simulink model "TZ"  (R2023a)
settings: Solver=VariableStepAuto  StartTime=0.0  StopTime=25.0  RelTol=1e-3
settings Model: Creator=zarok  LastModifiedBy=Georgiy

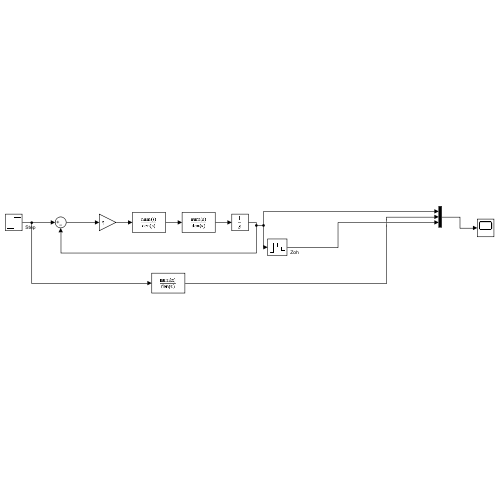
[thumbnail: Simulink's stored preview of the top-level diagram]
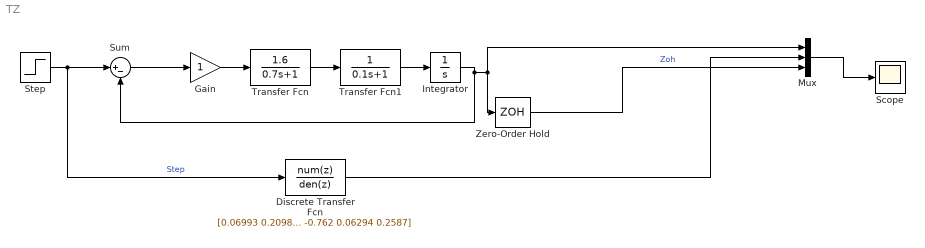
== system TZ ==
  Discrete Transfer Fcn : DiscreteTransferFcn  Numerator=[0.06993 0.2098 0.2098 0.06993]  Denominator=[1 -0.762 0.06294 0.2587]
  Gain : Gain
  Integrator : Integrator
  Mux : Mux  Inputs=3
  Scope : Scope
  Step : Step  SampleTime=0
  Sum : Sum  Inputs=|+-
  Transfer Fcn : TransferFcn  Numerator=[1.6]  Denominator=[0.7 1]
  Transfer Fcn1 : TransferFcn  Denominator=[0.1 1]
  Zero-Order Hold : ZeroOrderHold  SampleTime=-1
  wires:
  Mux/1 -> Scope/1
  Transfer Fcn/1 -> Transfer Fcn1/1
  Discrete Transfer Fcn/1 -> Mux/2
  Gain/1 -> Transfer Fcn/1
  Sum/1 -> Gain/1
  Transfer Fcn1/1 -> Integrator/1
  Step/1 -> Discrete Transfer Fcn/1, Sum/1  "Step"
  Integrator/1 -> Sum/2, Zero-Order Hold/1, Mux/1
  Zero-Order Hold/1 -> Mux/3  "Zoh"
